simulink model "intent"  (R2015b)
settings: Solver=ode4  StartTime=0.0  StopTime=inf  FixedStep=0.001  RelTol=1e-3
settings Model: Creator=KAREN  LastModifiedBy=KAREN

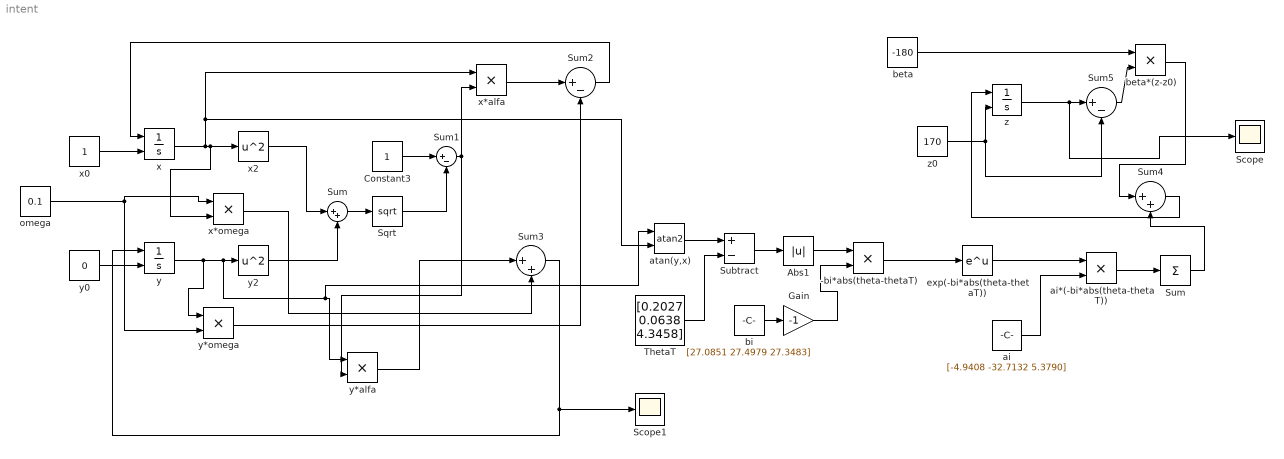
== system intent ==
  -bi*abs(theta-thetaT) : Product
  Abs1 : Abs
  Constant3 : Constant
  Gain : Gain  Gain=-1
  Scope : Scope
  Scope1 : Scope
  Sqrt : Sqrt  SaturateOnIntegerOverflow=on
  Subtract : Sum  Inputs=+-
  Sum : Sum  Inputs=|++
  "Sum " : Sum  Inputs=+
  Sum1 : Sum  Inputs=|+-
  Sum2 : Sum  Inputs=|+-
  Sum3 : Sum  Inputs=|++
  Sum4 : Sum  Inputs=|++
  Sum5 : Sum  Inputs=|+-
  ThetaT : Constant  Value=[0.2027 0.0638 4.3458]
  ai : Constant  Value=[-4.9408 -32.7132 5.3790]
  ai*(-bi*abs(theta-thetaT)) : Product
  atan(y,x) : Trigonometry  Operator=atan2
  beta : Constant  Value=-180
  beta*(z-z0) : Product
  bi : Constant  Value=[27.0851 27.4979 27.3483]
  exp(-bi*abs(theta-thetaT)) : Math  SaturateOnIntegerOverflow=on
  omega : Constant  Value=0.1
  x : Integrator  InitialConditionSource=external
  x*alfa : Product
  x*omega : Product
  x0 : Constant
  x2 : Math  Operator=square  SaturateOnIntegerOverflow=on
  y : Integrator  InitialConditionSource=external
  y*alfa : Product
  y*omega : Product
  y0 : Constant  Value=0
  y2 : Math  Operator=square  SaturateOnIntegerOverflow=on
  z : Integrator  InitialConditionSource=external
  z0 : Constant  Value=170
  wires:
  x0/1 -> x/2
  y0/1 -> y/2
  x/1 -> x*alfa/1, atan(y,x)/2, x*omega/2, x2/1
  x2/1 -> Sum/1
  y2/1 -> Sum/2
  Sum/1 -> Sqrt/1
  Sqrt/1 -> Sum1/2
  Constant3/1 -> Sum1/1
  omega/1 -> y*omega/2, x*omega/1
  Sum1/1 -> x*alfa/2, y*alfa/2
  y*omega/1 -> Sum2/2
  x*alfa/1 -> Sum2/1
  Sum2/1 -> x/1
  y*alfa/1 -> Sum3/1
  x*omega/1 -> Sum3/2
  Sum3/1 -> Scope1/1, y/1
  y/1 -> y*omega/1, atan(y,x)/1, y*alfa/1, y2/1
  atan(y,x)/1 -> Subtract/1
  ThetaT/1 -> Subtract/2
  Subtract/1 -> Abs1/1
  Abs1/1 -> -bi*abs(theta-thetaT)/1
  bi/1 -> Gain/1
  Gain/1 -> -bi*abs(theta-thetaT)/2
  -bi*abs(theta-thetaT)/1 -> exp(-bi*abs(theta-thetaT))/1
  exp(-bi*abs(theta-thetaT))/1 -> ai*(-bi*abs(theta-thetaT))/1
  ai/1 -> ai*(-bi*abs(theta-thetaT))/2
  ai*(-bi*abs(theta-thetaT))/1 -> "Sum "/1
  "Sum "/1 -> Sum4/2
  z0/1 -> Sum5/2, z/2
  beta/1 -> beta*(z-z0)/1
  z/1 -> Scope/1, Sum5/1
  Sum5/1 -> beta*(z-z0)/2
  beta*(z-z0)/1 -> Sum4/1
  Sum4/1 -> z/1
